simulink model "canrx_0x586"  (R2022b)
settings: Solver=VariableStepAuto  StartTime=0.0  StopTime=10.0  RelTol=1e-3
values from neighbouring files (symbols this model uses):
  K_CAN_GMLAN_RX_INVALID_SELECT = 0.0    [canrx_0x586.sldd]
  PLCANC_APCNTL_RQST_SEL_GMLAN = 1.0    [canrx_0x586.sldd]
  PLCANC_APCNTL_RQST_SEL_J1939 = 0.0    [canrx_0x586.sldd]
undefined symbols (not defined in the file or in its folder): K_CAN_GMLAN_RX_DEFAULT_GPS_ALTITUDE, K_CAN_GMLAN_RX_DEFAULT_GPS_ANTENNA_STAT, K_CAN_GMLAN_RX_DEFAULT_GPS_DIRECTION, K_CAN_GMLAN_RX_DEFAULT_GPS_HDOP, K_CAN_GMLAN_RX_DEFAULT_GPS_LATITUDE, K_CAN_GMLAN_RX_DEFAULT_GPS_LONGITUDE, K_CAN_GMLAN_RX_DEFAULT_GPS_SG_UB, K_CAN_GMLAN_RX_DEFAULT_GPS_TIME, K_CAN_GMLAN_RX_DEFAULT_GPS_VEH_SPEED, K_CAN_RQST_SEL_1, K_CAN_RQST_SEL_2, K_CAN_RX_SEL_2, K_RQST_DRCT_2
libraries: simulink x9
(part 2 of 2)

== system canrx_0x586/canrx_0x586_main/Select_Input_SYCANC_COM2AP_586_rx_gps_altitude ==
  can_invalid_can_rx_gps_altitude : Inport
  can_rx_gps_altitude : Inport  Port=2
  <initial=K_CAN_GMLAN_RX_DEFAULT_GPS_ALTITUDE> : UnitDelay  InitialCondition=K_CAN_GMLAN_RX_DEFAULT_GPS_ALTITUDE  SampleTime=-1  HasFrameUpgradeWarning=on
  K_CAN_RQST_SEL_1 : Constant  Value=K_CAN_RQST_SEL_1
  Multiport Switch : MultiPortSwitch  DataPortOrder=Zero-based contiguous  Inputs=5  zeroidx=on  SaturateOnIntegerOverflow=off  InputSameDT=off
  can_invalid_can_rqst_gps_altitude : Outport
  can_rqst_gps_altitude : Outport  Port=2
  wires:
  K_CAN_RQST_SEL_1/1 -> Multiport Switch/1
  <initial=K_CAN_GMLAN_RX_DEFAULT_GPS_ALTITUDE>/1 -> Multiport Switch/6, Multiport Switch/2, Multiport Switch/5
  Multiport Switch/1 -> can_rqst_gps_altitude/1, <initial=K_CAN_GMLAN_RX_DEFAULT_GPS_ALTITUDE>/1
  can_rx_gps_altitude/1 -> Multiport Switch/4, Multiport Switch/3
  can_invalid_can_rx_gps_altitude/1 -> can_invalid_can_rqst_gps_altitude/1

== system canrx_0x586/canrx_0x586_main/Select_Input_SYCANC_COM2AP_586_rx_gps_antenna_stat ==
  can_invalid_can_rx_gps_antenna_stat : Inport
  can_rx_gps_antenna_stat : Inport  Port=2
  <initial=K_CAN_GMLAN_RX_DEFAULT_GPS_ANTENNA_STAT> : UnitDelay  InitialCondition=K_CAN_GMLAN_RX_DEFAULT_GPS_ANTENNA_STAT  SampleTime=-1  HasFrameUpgradeWarning=on
  K_CAN_RQST_SEL_1 : Constant  Value=K_CAN_RQST_SEL_1
  Multiport Switch : MultiPortSwitch  DataPortOrder=Zero-based contiguous  Inputs=5  zeroidx=on  SaturateOnIntegerOverflow=off  InputSameDT=off
  can_invalid_can_rqst_gps_antenna_stat : Outport
  can_rqst_gps_antenna_stat : Outport  Port=2
  wires:
  K_CAN_RQST_SEL_1/1 -> Multiport Switch/1
  <initial=K_CAN_GMLAN_RX_DEFAULT_GPS_ANTENNA_STAT>/1 -> Multiport Switch/6, Multiport Switch/2, Multiport Switch/5
  Multiport Switch/1 -> can_rqst_gps_antenna_stat/1, <initial=K_CAN_GMLAN_RX_DEFAULT_GPS_ANTENNA_STAT>/1
  can_rx_gps_antenna_stat/1 -> Multiport Switch/4, Multiport Switch/3
  can_invalid_can_rx_gps_antenna_stat/1 -> can_invalid_can_rqst_gps_antenna_stat/1

== system canrx_0x586/canrx_0x586_main/Select_Input_SYCANC_COM2AP_586_rx_gps_direction ==
  can_invalid_can_rx_gps_direction : Inport
  can_rx_gps_direction : Inport  Port=2
  <initial=K_CAN_J_RX_INIT_XXX> : UnitDelay  SampleTime=-1  HasFrameUpgradeWarning=on
  K_CAN_RQST_SEL_2 : Constant  Value=K_CAN_RQST_SEL_2
  K_RQST_DRCT_2 : Constant  Value=K_RQST_DRCT_2
  Multiport Switch : MultiPortSwitch  DataPortOrder=Zero-based contiguous  Inputs=5  zeroidx=on  SaturateOnIntegerOverflow=off  InputSameDT=off
  can_invalid_can_rqst_gps_direction : Outport
  can_rqst_gps_direction : Outport  Port=2
  wires:
  K_CAN_RQST_SEL_2/1 -> Multiport Switch/1
  <initial=K_CAN_J_RX_INIT_XXX>/1 -> Multiport Switch/6, Multiport Switch/5
  Multiport Switch/1 -> can_rqst_gps_direction/1, <initial=K_CAN_J_RX_INIT_XXX>/1
  can_rx_gps_direction/1 -> Multiport Switch/4, Multiport Switch/3
  K_RQST_DRCT_2/1 -> Multiport Switch/2
  can_invalid_can_rx_gps_direction/1 -> can_invalid_can_rqst_gps_direction/1

== system canrx_0x586/canrx_0x586_main/Select_Input_SYCANC_COM2AP_586_rx_gps_hdop ==
  can_invalid_can_rx_gps_hdop : Inport
  can_rx_gps_hdop : Inport  Port=2
  <initial=K_CAN_J_RX_INIT_XXX> : UnitDelay  SampleTime=-1  HasFrameUpgradeWarning=on
  K_CAN_RQST_SEL_2 : Constant  Value=K_CAN_RQST_SEL_2
  K_RQST_DRCT_2 : Constant  Value=K_RQST_DRCT_2
  Multiport Switch : MultiPortSwitch  DataPortOrder=Zero-based contiguous  Inputs=5  zeroidx=on  SaturateOnIntegerOverflow=off  InputSameDT=off
  can_invalid_can_rqst_gps_hdop : Outport
  can_rqst_gps_hdop : Outport  Port=2
  wires:
  K_CAN_RQST_SEL_2/1 -> Multiport Switch/1
  <initial=K_CAN_J_RX_INIT_XXX>/1 -> Multiport Switch/6, Multiport Switch/5
  Multiport Switch/1 -> can_rqst_gps_hdop/1, <initial=K_CAN_J_RX_INIT_XXX>/1
  can_rx_gps_hdop/1 -> Multiport Switch/4, Multiport Switch/3
  K_RQST_DRCT_2/1 -> Multiport Switch/2
  can_invalid_can_rx_gps_hdop/1 -> can_invalid_can_rqst_gps_hdop/1

== system canrx_0x586/canrx_0x586_main/Select_Input_SYCANC_COM2AP_586_rx_gps_latitude ==
  can_invalid_can_rx_gps_latitude : Inport
  can_rx_gps_latitude : Inport  Port=2
  <initial=K_CAN_J_RX_INIT_XXX> : UnitDelay  SampleTime=-1  HasFrameUpgradeWarning=on
  K_CAN_RQST_SEL_2 : Constant  Value=K_CAN_RQST_SEL_2
  K_RQST_DRCT_2 : Constant  Value=K_RQST_DRCT_2
  Multiport Switch : MultiPortSwitch  DataPortOrder=Zero-based contiguous  Inputs=5  zeroidx=on  SaturateOnIntegerOverflow=off  InputSameDT=off
  can_invalid_can_rqst_gps_latitude : Outport
  can_rqst_gps_latitude : Outport  Port=2
  wires:
  K_CAN_RQST_SEL_2/1 -> Multiport Switch/1
  <initial=K_CAN_J_RX_INIT_XXX>/1 -> Multiport Switch/6, Multiport Switch/5
  Multiport Switch/1 -> can_rqst_gps_latitude/1, <initial=K_CAN_J_RX_INIT_XXX>/1
  can_rx_gps_latitude/1 -> Multiport Switch/4, Multiport Switch/3
  K_RQST_DRCT_2/1 -> Multiport Switch/2
  can_invalid_can_rx_gps_latitude/1 -> can_invalid_can_rqst_gps_latitude/1

== system canrx_0x586/canrx_0x586_main/Select_Input_SYCANC_COM2AP_586_rx_gps_longitude ==
  can_invalid_can_rx_gps_longitude : Inport
  can_rx_gps_longitude : Inport  Port=2
  can_invalid_can_rqst_gps_longitude : Outport
  can_rqst_gps_longitude : Outport  Port=2
  wires:
  can_invalid_can_rx_gps_longitude/1 -> can_invalid_can_rqst_gps_longitude/1
  can_rx_gps_longitude/1 -> can_rqst_gps_longitude/1

== system canrx_0x586/canrx_0x586_main/Select_Input_SYCANC_COM2AP_586_rx_gps_sg_ub ==
  can_invalid_can_rx_gps_sg_ub : Inport
  can_rx_gps_sg_ub : Inport  Port=2
  <initial=K_CAN_GMLAN_RX_DEFAULT_GPS_SG_UB> : UnitDelay  InitialCondition=K_CAN_GMLAN_RX_DEFAULT_GPS_SG_UB  SampleTime=-1  HasFrameUpgradeWarning=on
  K_CAN_RQST_SEL_1 : Constant  Value=K_CAN_RQST_SEL_1
  Multiport Switch : MultiPortSwitch  DataPortOrder=Zero-based contiguous  Inputs=5  zeroidx=on  SaturateOnIntegerOverflow=off  InputSameDT=off
  can_invalid_can_rqst_gps_sg_ub : Outport
  can_rqst_gps_sg_ub : Outport  Port=2
  wires:
  K_CAN_RQST_SEL_1/1 -> Multiport Switch/1
  <initial=K_CAN_GMLAN_RX_DEFAULT_GPS_SG_UB>/1 -> Multiport Switch/6, Multiport Switch/2, Multiport Switch/5
  Multiport Switch/1 -> can_rqst_gps_sg_ub/1, <initial=K_CAN_GMLAN_RX_DEFAULT_GPS_SG_UB>/1
  can_rx_gps_sg_ub/1 -> Multiport Switch/4, Multiport Switch/3
  can_invalid_can_rx_gps_sg_ub/1 -> can_invalid_can_rqst_gps_sg_ub/1

== system canrx_0x586/canrx_0x586_main/Select_Input_SYCANC_COM2AP_586_rx_gps_time ==
  can_invalid_can_rx_gps_time : Inport
  can_rx_gps_time : Inport  Port=2
  can_invalid_can_rqst_gps_time : Outport
  can_rqst_gps_time : Outport  Port=2
  wires:
  can_invalid_can_rx_gps_time/1 -> can_invalid_can_rqst_gps_time/1
  can_rx_gps_time/1 -> can_rqst_gps_time/1

== system canrx_0x586/canrx_0x586_main/Select_Input_SYCANC_COM2AP_586_rx_gps_veh_speed ==
  can_invalid_can_rx_gps_veh_speed : Inport
  can_rx_gps_veh_speed : Inport  Port=2
  can_invalid_can_rqst_gps_veh_speed : Outport
  can_rqst_gps_veh_speed : Outport  Port=2
  wires:
  can_invalid_can_rx_gps_veh_speed/1 -> can_invalid_can_rqst_gps_veh_speed/1
  can_rx_gps_veh_speed/1 -> can_rqst_gps_veh_speed/1
